simulink model "test_samplecount"  (Simulink 6.5)
settings: Solver=VariableStepDiscrete  StartTime=0.0  StopTime=400  RelTol=1e-3
undefined symbols (not defined in the file or in its folder): sigbuilder_block
libraries: xbsIndex_r4 x9, nort_sysgenlib x1
settings Model: Creator=nort  LastModifiedBy=nort

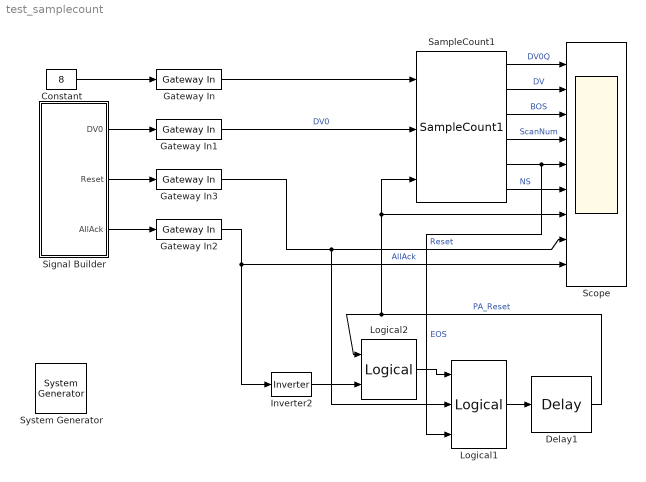
== system test_samplecount ==
  " System Generator" : xbsIndex_r4/ System Generator  Tag=genX  SystemSampleTime=-1  xilinxfamily=virtex4  part=xc4vsx35  speed=-10  package=ff668  synthesis_tool=XST  directory=./netlist  testbench=off  simulink_period=1  sysclk_period=10  incr_netlist=off  trim_vbits=Everywhere in SubSystem  dbl_ovrd=According to Block Masks  core_generation=According to Block Masks  run_coregen=off  deprecated_control=off  eval_field=0  block_type=sysgen
      settings: block_version=9.2.01
  Constant : Constant  Value=8  OutDataType=sfix(16)  ConRadixGroup=Use specified scaling  OutScaling=2^0  SampleTime=inf  FramePeriod=inf
  Delay1 : xbsIndex_r4/Delay  en=off  latency=1  dbl_ovrd=off  reg_retiming=off  block_type=delay
      settings: block_version=9.2.01
  Gateway In : xbsIndex_r4/Gateway In  arith_type=Unsigned  n_bits=12  bin_pt=0  quantization="Round  (unbiased: +/- Inf)"  overflow=Saturate  period=1  dbl_ovrd=off  timing_constraint=None  locs_specified=off  LOCs={}  block_type=gatewayin
      settings: infoedit="Gateway in block.  Converts inputs of type Simulink integer, double and fixed point to  Xilinx fixed point type.<P><P>Hardware notes:  In hardware these blocks become top level input ports."  block_version=9.2.01
  Gateway In1 : xbsIndex_r4/Gateway In  arith_type=Boolean  n_bits=12  bin_pt=0  quantization="Round  (unbiased: +/- Inf)"  overflow=Saturate  period=1  dbl_ovrd=off  timing_constraint=None  locs_specified=off  LOCs={}  block_type=gatewayin
      settings: infoedit="Gateway in block.  Converts inputs of type Simulink integer, double and fixed point to  Xilinx fixed point type.<P><P>Hardware notes:  In hardware these blocks become top level input ports."  block_version=9.2.01
  Gateway In2 : xbsIndex_r4/Gateway In  arith_type=Boolean  n_bits=12  bin_pt=0  quantization="Round  (unbiased: +/- Inf)"  overflow=Saturate  period=1  dbl_ovrd=off  timing_constraint=None  locs_specified=off  LOCs={}  block_type=gatewayin
      settings: infoedit="Gateway in block.  Converts inputs of type Simulink integer, double and fixed point to  Xilinx fixed point type.<P><P>Hardware notes:  In hardware these blocks become top level input ports."  block_version=9.2.01
  Gateway In3 : xbsIndex_r4/Gateway In  arith_type=Boolean  n_bits=12  bin_pt=0  quantization="Round  (unbiased: +/- Inf)"  overflow=Saturate  period=1  dbl_ovrd=off  timing_constraint=None  locs_specified=off  LOCs={}  block_type=gatewayin
      settings: infoedit="Gateway in block.  Converts inputs of type Simulink integer, double and fixed point to  Xilinx fixed point type.<P><P>Hardware notes:  In hardware these blocks become top level input ports."  block_version=9.2.01
  Inverter2 : xbsIndex_r4/Inverter  en=off  latency=0  dbl_ovrd=off  block_type=inv
      settings: block_version=9.2.01
  Logical1 : xbsIndex_r4/Logical  logical_function=OR  inputs=3  en=off  latency=0  precision=Full  arith_type=Unsigned  n_bits=16  bin_pt=0  align_bp=on  dbl_ovrd=off  block_type=logical
      settings: block_version=9.2.01
  Logical2 : xbsIndex_r4/Logical  logical_function=AND  inputs=2  en=off  latency=0  precision=Full  arith_type=Unsigned  n_bits=16  bin_pt=0  align_bp=on  dbl_ovrd=off  block_type=logical
      settings: block_version=9.2.01
  SampleCount1 : nort_sysgenlib/SampleCount1  SystemSampleTime=-1
  Scope : Scope  NumInputPorts=9
      settings: TimeRange=400  YMin=-0.25~-0.25~-0.25~-5~-0.25~-0.25~-0.25~-0.25~-0.25  YMax=1.25~1.25~1.25~5~1.25~10~1.25~1.25~1.25
  Signal Builder : Subsystem  Tag=STV Subsys  LoadFcn=sigbuilder_block('load',[160.5 98.25 550.5 399.75 ]);  StartFcn=sigbuilder_block('start');  StopFcn=sigbuilder_block('stop');  ClipboardFcn=sigbuilder_block('clipboard');  mask(Sigbuilder block){}
      mask help: Sigbuilder GUI
      mask init:
      | if ~strcmp(get_param(bdroot(gcbh),'SimulationStatus'),'stopped') tuvar = sigbuilder_block('maskInit'); end
      settings: CopyFcn=sigbuilder_block('copy');  DeleteFcn=sigbuilder_block('delete');  ModelCloseFcn=sigbuilder_block('modelClose');  PreSaveFcn=sigbuilder_block('preSave');  NameChangeFcn=sigbuilder_block('namechange');  OpenFcn=sigbuilder_block('open',[437.6 199.2 550.4 400 ]);  CloseFcn=sigbuilder_block('close');
      mask Display: plot(0,0,100,100,[10,10,40,40,10],[80,20,20,80,80],[40,10],[50,50], [40,27,10],[65,72,56],[40,25,25,10],[28,28,43,43]);
  wires:
  Gateway In/1 -> SampleCount1/1
  Constant/1 -> Gateway In/1
  Gateway In1/1 -> SampleCount1/2  "DV0"
  Gateway In3/1 -> Scope/8, Logical1/2  "Reset"
  SampleCount1/3 -> Scope/3  "BOS"
  SampleCount1/1 -> Scope/1  "DV0Q"
  SampleCount1/2 -> Scope/2  "DV"
  SampleCount1/6 -> Scope/6  "NS"
  SampleCount1/5 -> Scope/5, Logical1/3  "EOS"
  SampleCount1/4 -> Scope/4  "ScanNum"
  Signal Builder/2(Reset) -> Gateway In3/1
  Signal Builder/1(DV0) -> Gateway In1/1
  Logical2/1 -> Logical1/1
  Logical1/1 -> Delay1/1
  Inverter2/1 -> Logical2/2
  Delay1/1 -> Logical2/1, SampleCount1/3, Scope/7  "PA_Reset"
  Signal Builder/3(AllAck) -> Gateway In2/1
  Gateway In2/1 -> Inverter2/1, Scope/9  "AllAck"

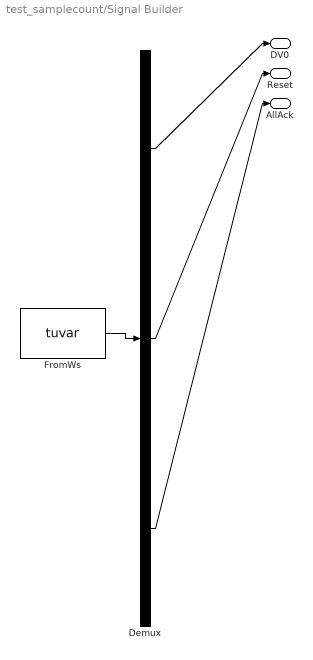
== system test_samplecount/Signal Builder ==
  Demux : Demux  Tag=STV Demux  Outputs=3
  FromWs : FromWorkspace  Tag=STV FromWs  VariableName=tuvar  SampleTime=0  SigBuilderData=DataTag1  VnvData=DataTag2
      SigBuilderData=|
      | channels(1).label = 'DV0'
      | channels(1).allXData{1} = [0 1 1 4 4 5 5 8 8 9 9 12 12 13 13 16 16 17 17 20 20 21 21 24 24 25 25 28 28 29 29 32 32 33 33 36 36 37 37 40 40 41 41 44 44 45 45 48 48 49 49 52 52 53 53 56 56 57 57 60 60 61 61 64 64 65 65 68 68 69 69 72 72 73 73 76 76 77 77 80 80 81 81 84 84 85 85 88 88 89 89 92 92 93 93 96 96 97 97 100 100 101 101 104 104 105 105 108 108 109 109 112 112 113 113 116 116 117 117 120 120 121 121 124 124 125 125 128 128 129 129 132 132 133 133 136 136 137 137 140 140 141 141 144 144 145 145 148 148 149 149 152 152 153 153 156 156 157 157 160 160 161 161 164 164 165 165 168 168 169 169 172 172 173 173 176 176 177 177 180 180 181 181 184 184 185 185 188 188 189 189 192 192 193 193 196 196 197 197 200 200 201 201 204 204 205 205 208 208 209 209 212 212 213 213 216 216 217 217 220 220 221 221 224 224 225 225 228 228 229 229 232 232 233 233 236 236 237 237 240 240 241 241 244 244 245 245 248 248 249 249 252 252 253 253 256 256 257 257 260 260 261 261 264 264 265 265 268 268 269 269 272 272 273 273 276 276 277 277 280 280 281 281 284 284 285 285 288 288 289 289 292 292 293 293 296 296 297 297 300 300 301 301 304 304 305 305 308 308 309 309 312 312 313 313 316 316 317 317 320 320 321 321 324 324 325 325 328 328 329 329 332 332 333 333 336 336 337 337 340 340 341 341 344 344 345 345 348 348 349 349 352 352 353 353 356 356 357 357 360 360 361 361 364 364 365 365 368 368 369 369 372 372 373 373 376 376 377 377 380 380 381 381 384 384 385 385 388 388 389 389 392 392 393 393 396 396 397 397 400]
      | channels(1).allXData{2} = [0 1 1 4 4 5 5 8 8 9 9 12 12 13 13 16 16 17 17 20 20 21 21 24 24 25 25 28 28 29 29 32 32 33 33 36 36 37 37 40 40 41 41 44 44 45 45 48 48 49 49 52 52 53 53 56 56 57 57 60 60 61 61 64 64 65 65 68 68 69 69 72 72 73 73 76 76 77 77 80 80 81 81 84 84 85 85 88 88 89 89 92 92 93 93 96 96 97 97 100 100 101 101 104 104 105 105 108 108 109 109 112 112 113 113 116 116 117 117 120 120 121 121 124 124 125 125 128 128 129 129 132 132 133 133 136 136 137 137 140 140 141 141 144 144 145 145 148 148 149 149 152 152 153 153 156 156 157 157 160 160 161 161 164 164 165 165 168 168 169 169 172 172 173 173 176 176 177 177 180 180 181 181 184 184 185 185 188 188 189 189 192 192 193 193 196 196 197 197 200 200 201 201 204 204 205 205 208 208 209 209 212 212 213 213 216 216 217 217 220 220 221 221 224 224 225 225 228 228 229 229 232 232 233 233 236 236 237 237 240 240 241 241 244 244 245 245 248 248 249 249 252 252 253 253 256 256 257 257 260 260 261 261 264 264 265 265 268 268 269 269 272 272 273 273 276 276 277 277 280 280 281 281 284 284 285 285 288 288 289 289 292 292 293 293 296 296 297 297 300 300 301 301 304 304 305 305 308 308 309 309 312 312 313 313 316 316 317 317 320 320 321 321 324 324 325 325 328 328 329 329 332 332 333 333 336 336 337 337 340 340 341 341 344 344 345 345 348 348 349 349 352 352 353 353 356 356 357 357 360 360 361 361 364 364 365 365 368 368 369 369 372 372 373 373 376 376 377 377 380 380 381 381 384 384 385 385 388 388 389 389 392 392 393 393 396 396 397 397 400]
      | channels(1).allXData{3} = [0 1 1 4 4 5 5 8 8 9 9 12 12 13 13 16 16 17 17 20 20 21 21 24 24 25 25 28 28 29 29 32 32 33 33 36 36 37 37 40 40 41 41 44 44 45 45 48 48 49 49 52 52 53 53 56 56 57 57 60 60 61 61 64 64 65 65 68 68 69 69 72 72 73 73 76 76 77 77 80 80 81 81 84 84 85 85 88 88 89 89 92 92 93 93 96 96 97 97 100 100 101 101 104 104 105 105 108 108 109 109 112 112 113 113 116 116 117 117 120 120 121 121 124 124 125 125 128 128 129 129 132 132 133 133 136 136 137 137 140 140 141 141 144 144 145 145 148 148 149 149 152 152 153 153 156 156 157 157 160 160 161 161 164 164 165 165 168 168 169 169 172 172 173 173 176 176 177 177 180 180 181 181 184 184 185 185 188 188 189 189 192 192 193 193 196 196 197 197 200 200 201 201 204 204 205 205 208 208 209 209 212 212 213 213 216 216 217 217 220 220 221 221 224 224 225 225 228 228 229 229 232 232 233 233 236 236 237 237 240 240 241 241 244 244 245 245 248 248 249 249 252 252 253 253 256 256 257 257 260 260 261 261 264 264 265 265 268 268 269 269 272 272 273 273 276 276 277 277 280 280 281 281 284 284 285 285 288 288 289 289 292 292 293 293 296 296 297 297 300 300 301 301 304 304 305 305 308 308 309 309 312 312 313 313 316 316 317 317 320 320 321 321 324 324 325 325 328 328 329 329 332 332 333 333 336 336 337 337 340 340 341 341 344 344 345 345 348 348 349 349 352 352 353 353 356 356 357 357 360 360 361 361 364 364 365 365 368 368 369 369 372 372 373 373 376 376 377 377 380 380 381 381 384 384 385 385 388 388 389 389 392 392 393 393 396 396 397 397 400]
      | channels(1).allYData{1} = [1 1 0 0 1 1 0 0 1 1 0 0 1 1 0 0 1 1 0 0 1 1 0 0 1 1 0 0 1 1 0 0 1 1 0 0 1 1 0 0 1 1 0 0 1 1 0 0 1 1 0 0 1 1 0 0 1 1 0 0 1 1 0 0 1 1 0 0 1 1 0 0 1 1 0 0 1 1 0 0 1 1 0 0 1 1 0 0 1 1 0 0 1 1 0 0 1 1 0 0 1 1 0 0 1 1 0 0 1 1 0 0 1 1 0 0 1 1 0 0 1 1 0 0 1 1 0 0 1 1 0 0 1 1 0 0 1 1 0 0 1 1 0 0 1 1 0 0 1 1 0 0 1 1 0 0 1 1 0 0 1 1 0 0 1 1 0 0 1 1 0 0 1 1 0 0 1 1 0 0 1 1 0 0 1 1 0 0 1 1 0 0 1 1 0 0 1 1 0 0 1 1 0 0 1 1 0 0 1 1 0 0 1 1 0 0 1 1 0 0 1 1 0 0 1 1 0 0 1 1 0 0 1 1 0 0 1 1 0 0 1 1 0 0 1 1 0 0 1 1 0 0 1 1 0 0 1 1 0 0 1 1 0 0 1 1 0 0 1 1 0 0 1 1 0 0 1 1 0 0 1 1 0 0 1 1 0 0 1 1 0 0 1 1 0 0 1 1 0 0 1 1 0 0 1 1 0 0 1 1 0 0 1 1 0 0 1 1 0 0 1 1 0 0 1 1 0 0 1 1 0 0 1 1 0 0 1 1 0 0 1 1 0 0 1 1 0 0 1 1 0 0 1 1 0 0 1 1 0 0 1 1 0 0 1 1 0 0 1 1 0 0 1 1 0 0 1 1 0 0 1 1 0 0 1 1 0 0 1 1 0 0 1 1 0 0 1 1 0 0]
      | channels(1).allYData{2} = [1 1 0 0 1 1 0 0 1 1 0 0 1 1 0 0 1 1 0 0 1 1 0 0 1 1 0 0 1 1 0 0 1 1 0 0 1 1 0 0 1 1 0 0 1 1 0 0 1 1 0 0 1 1 0 0 1 1 0 0 1 1 0 0 1 1 0 0 1 1 0 0 1 1 0 0 1 1 0 0 1 1 0 0 1 1 0 0 1 1 0 0 1 1 0 0 1 1 0 0 1 1 0 0 1 1 0 0 1 1 0 0 1 1 0 0 1 1 0 0 1 1 0 0 1 1 0 0 1 1 0 0 1 1 0 0 1 1 0 0 1 1 0 0 1 1 0 0 1 1 0 0 1 1 0 0 1 1 0 0 1 1 0 0 1 1 0 0 1 1 0 0 1 1 0 0 1 1 0 0 1 1 0 0 1 1 0 0 1 1 0 0 1 1 0 0 1 1 0 0 1 1 0 0 1 1 0 0 1 1 0 0 1 1 0 0 1 1 0 0 1 1 0 0 1 1 0 0 1 1 0 0 1 1 0 0 1 1 0 0 1 1 0 0 1 1 0 0 1 1 0 0 1 1 0 0 1 1 0 0 1 1 0 0 1 1 0 0 1 1 0 0 1 1 0 0 1 1 0 0 1 1 0 0 1 1 0 0 1 1 0 0 1 1 0 0 1 1 0 0 1 1 0 0 1 1 0 0 1 1 0 0 1 1 0 0 1 1 0 0 1 1 0 0 1 1 0 0 1 1 0 0 1 1 0 0 1 1 0 0 1 1 0 0 1 1 0 0 1 1 0 0 1 1 0 0 1 1 0 0 1 1 0 0 1 1 0 0 1 1 0 0 1 1 0 0 1 1 0 0 1 1 0 0 1 1 0 0 1 1 0 0 1 1 0 0 1 1 0 0]
      | channels(1).allYData{3} = [1 1 0 0 1 1 0 0 1 1 0 0 1 1 0 0 1 1 0 0 1 1 0 0 1 1 0 0 1 1 0 0 1 1 0 0 1 1 0 0 1 1 0 0 1 1 0 0 1 1 0 0 1 1 0 0 1 1 0 0 1 1 0 0 1 1 0 0 1 1 0 0 1 1 0 0 1 1 0 0 1 1 0 0 1 1 0 0 1 1 0 0 1 1 0 0 1 1 0 0 1 1 0 0 1 1 0 0 1 1 0 0 1 1 0 0 1 1 0 0 1 1 0 0 1 1 0 0 1 1 0 0 1 1 0 0 1 1 0 0 1 1 0 0 1 1 0 0 1 1 0 0 1 1 0 0 1 1 0 0 1 1 0 0 1 1 0 0 1 1 0 0 1 1 0 0 1 1 0 0 1 1 0 0 1 1 0 0 1 1 0 0 1 1 0 0 1 1 0 0 1 1 0 0 1 1 0 0 1 1 0 0 1 1 0 0 1 1 0 0 1 1 0 0 1 1 0 0 1 1 0 0 1 1 0 0 1 1 0 0 1 1 0 0 1 1 0 0 1 1 0 0 1 1 0 0 1 1 0 0 1 1 0 0 1 1 0 0 1 1 0 0 1 1 0 0 1 1 0 0 1 1 0 0 1 1 0 0 1 1 0 0 1 1 0 0 1 1 0 0 1 1 0 0 1 1 0 0 1 1 0 0 1 1 0 0 1 1 0 0 1 1 0 0 1 1 0 0 1 1 0 0 1 1 0 0 1 1 0 0 1 1 0 0 1 1 0 0 1 1 0 0 1 1 0 0 1 1 0 0 1 1 0 0 1 1 0 0 1 1 0 0 1 1 0 0 1 1 0 0 1 1 0 0 1 1 0 0 1 1 0 0 1 1 0 0 1 1 0 0]
      | channels(2).label = 'Reset'
      | channels(2).allXData = {[0 10 10 400], [0 10 10 400], [0 10 10 400]}
      | channels(2).allYData = {[1 1 0 0], [1 1 0 0], [1 1 0 0]}
      | channels(3).label = 'AllAck'
      | channels(3).allXData = {[0 7 7 18 18 42 42 58 58 400], [0 7 7 18 18 43 43 58 58 400], [0 7 7 18 18 44 44 58 58 400]}
      | channels(3).allYData = {[0 0 1 1 0 0 1 1 0 0], [0 0 1 1 0 0 1 1 0 0], [0 0 1 1 0 0 1 1 0 0]}
      | common.afterFinalStr = 'Extrapolate'
      | common.sampleTime = 0
      | dataSet(1).timeRange = [0 400]
      | dataSet(1).name = 'Group 1'
      | dataSet(2).timeRange = [0 400]
      | dataSet(2).name = 'Group 2'
      | dataSet(3).timeRange = [0 400]
      | dataSet(3).name = 'Group 3'
  DV0 : Outport  Tag=STV Outport
  Reset : Outport  Tag=STV Outport  Port=2
  AllAck : Outport  Tag=STV Outport  Port=3
  wires:
  FromWs/1 -> Demux/1
  Demux/1 -> DV0/1
  Demux/2 -> Reset/1
  Demux/3 -> AllAck/1
